simulink model "MicrowaveModified"  (Simulink 8.7)
settings: Solver=ode45  StartTime=0.0  StopTime=20  RelTol=1e-3
settings Model: Creator=bourbouh  LastModifiedBy=bourbouh
settings DataIOCC: SaveFormat=Dataset
settings DebuggingCC: UnderspecifiedInitializationDetection=Simplified  MergeDetectMultiDrivingBlocksExec=error

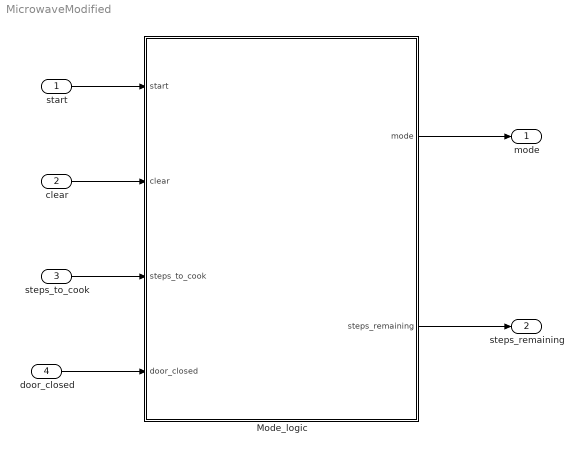
== system MicrowaveModified ==
  start : Inport
  clear : Inport  Port=2
  steps_to_cook : Inport  Port=3
  door_closed : Inport  Port=4
  Mode_logic : Stateflow chart  TreatAsAtomicUnit=on
  mode : Outport
  steps_remaining : Outport  Port=2
  wires:
  start/1 -> Mode_logic/1(start)
  door_closed/1 -> Mode_logic/4(door_closed)
  steps_to_cook/1 -> Mode_logic/3(steps_to_cook)
  clear/1 -> Mode_logic/2(clear)
  Mode_logic/1(mode) -> mode/1
  Mode_logic/2(steps_remaining) -> steps_remaining/1

== stateflow chart Mode_logic ==
  settings: updateMethod=DISCRETE  sampleTime=1
  state SETUP
    entry:
    mode=1;
    steps_remaining = steps_to_cook;
  state RUNNING
    state COOKING
      entry: mode=2;
    state SUSPENDED
      entry: mode=3;
    COOKING -> COOKING [order 2] : [steps_remaining > 0]
        | /steps_remaining--;
    (default) -> (junction 7)
    (junction 7) -> COOKING [order 1] : [door_closed]
    (junction 7) -> SUSPENDED [order 2]
    SUSPENDED -> COOKING [order 2] : [start && ...
        | door_closed]
    COOKING -> SUSPENDED [order 1] : [clear || ...
        | !door_closed]
  (default) -> SETUP
  SETUP -> RUNNING : [start && steps_to_cook > 0]{steps_remaining = steps_to_cook;}
  (junction 20) -> SETUP
  RUNNING -> (junction 20) : [steps_remaining <= 0]
  SUSPENDED -> (junction 20) [order 1] : [clear]
  data: start input boolean; clear input boolean; steps_to_cook input uint16; door_closed input boolean; mode output uint8; steps_remaining output uint16 [0..600]
